simulink model "space_state_model"  (R2018a)
settings: Solver=ode45  StartTime=0.0  StopTime=ttotal  MaxStep=1e-2  RelTol=1e-8  EnableMultiTasking=on
values from neighbouring files (symbols this model uses):
  A = [0 1 ; a1 a2]    [e_12.m]    (also in e_13.m; e_8.m; e_9.m; lab3.m)
  B = [0;  1/J]    [e_12.m]    (also in e_13.m; e_8.m; e_9.m; lab3.m)
  C = [1 0]    [e_12.m]    (also in e_13.m = [1 0; 0 1]; e_8.m = [1 0; 0 1]; e_9.m = [1 0; 0 1]; lab3.m = [1 0; 0 1])
  D = [0]    [e_12.m]    (also in e_13.m = [ 0; 0]; e_8.m = [ 0; 0]; e_9.m = [ 0; 0]; lab3.m = [ 0; 0])
  J = ((M*L^2)/3) + (m * l(n)^2)    [e_12.m]    (also in e_13.m = M*L^2/3+m_s*l^2; e_8.m = 0.0445; e_9.m = ((M*L^2)/3) + (m * l^2); lab3.m = M*L^2/3+m_s*l^2)
  T = T_v(n)    [e_11.m]    (also in e_13.m = 0; e_8.m = 0; e_9.m = 0; lab3.m = 0)
  x0 = [pi/4 0]    [e_13.m]    (also in e_8.m = vec_prop(:,n); e_9.m; lab3.m; lab3_1.m = [0 pi/4])
settings Model: Creator=ricar  LastModifiedBy=root
settings DataIOCC: SaveFormat=Array
settings OptimizationCC: LifeSpan=inf
settings DebuggingCC: SFUnexpectedBacktrackingDiag=warning  SFNoUnconditionalDefaultTransitionDiag=warning  SFExecutionAtInitializationDiag=none
settings CodeAppCC: StateflowObjectComments=on
settings GRTTargetCC: TargetLangStandard=C89/C90 (ANSI)  GeneratePreprocessorConditionals=Disable all
settings ConfigComp: CovMetricSettings=dw  CovHtmlReporting=on  CovSaveCumulativeToWorkspaceVar=on  CovSaveSingleToWorkspaceVar=on  CovExternalEMLEnable=off

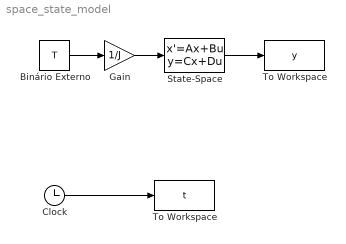
== system space_state_model ==
  Binário Externo : Constant  Value=T
  Clock : Clock
  Gain : Gain  Gain=1/J
  State-Space : StateSpace  A=A  B=B  C=C  D=D  InitialCondition=x0  ContinuousStateAttributes='Tethas'
  To Workspace : ToWorkspace  VariableName=y  SampleTime=-1
  "To Workspace " : ToWorkspace  VariableName=t  SampleTime=-1
  wires:
  Binário Externo/1 -> Gain/1
  Gain/1 -> State-Space/1
  State-Space/1 -> To Workspace/1
  Clock/1 -> "To Workspace "/1
